simulink model "part2"  (R2020a)
settings: Solver=ode23t  StartTime=0.0  StopTime=10  FixedStep=0.001  MaxStep=0.001  RelTol=1e-20
values from neighbouring files (symbols this model uses):
  mu = 1/82.45    (= 0.0121285627653)    [part1_sim.m]
  mu_star = 1 - mu    (= 0.987871437235)    [part1_sim.m]
settings Model: Creator=Ataka  LastModifiedBy=Ataka

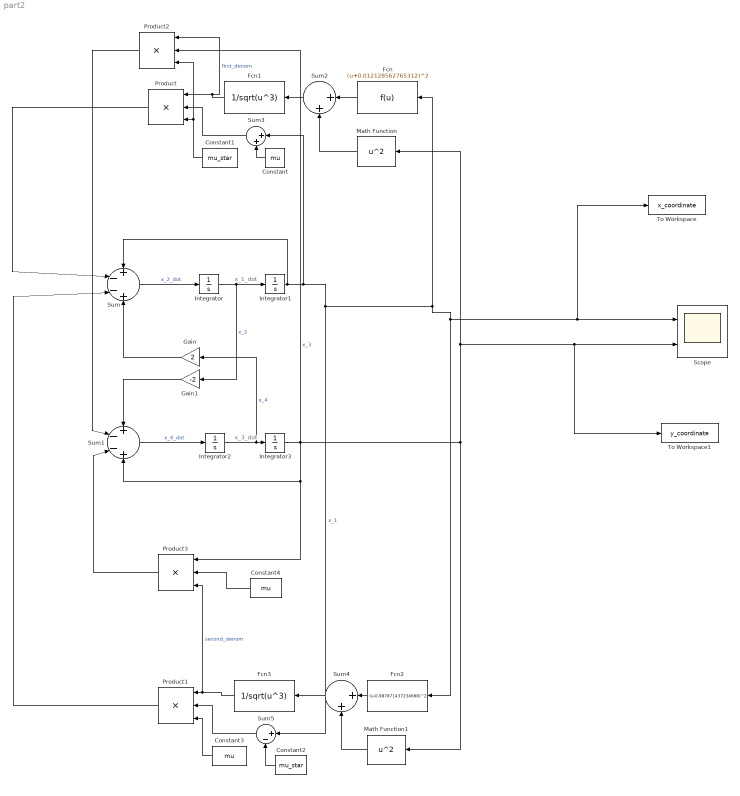
== system part2 ==
  note: x_1_dot
  note: x_3_dot
  Constant : Constant  Value=mu
  Constant1 : Constant  Value=mu_star
  Constant2 : Constant  Value=mu_star
  Constant3 : Constant  Value=mu
  Constant4 : Constant  Value=mu
  Fcn : Fcn  Expr=(u+0.012128562765312)^2
  Fcn1 : Fcn  Expr=1/sqrt(u^3)
  Fcn2 : Fcn  Expr=(u-0.987871437234688)^2
  Fcn3 : Fcn  Expr=1/sqrt(u^3)
  Gain : Gain  Gain=2
  Gain1 : Gain  Gain=-2
  Integrator : Integrator
  Integrator1 : Integrator  InitialCondition=1.2
  Integrator2 : Integrator  InitialCondition=-1.0494
  Integrator3 : Integrator
  Math Function : Math  Operator=square  SaturateOnIntegerOverflow=on
  Math Function1 : Math  Operator=square  SaturateOnIntegerOverflow=on
  Product{,1..3} (4 alike) : Product  Inputs=3
  Scope : Scope  NumInputPorts=2
  Sum : Sum  Inputs=+--+
  Sum1 : Sum  Inputs=+--+
  Sum2 : Sum  Inputs=|++
  Sum3 : Sum  Inputs=|++
  Sum4 : Sum  Inputs=|++
  Sum5 : Sum  Inputs=|+-
  To Workspace : ToWorkspace  VariableName=x_coordinate  SaveFormat=Timeseries  SampleTime=-1
  To Workspace1 : ToWorkspace  VariableName=y_coordinate  SaveFormat=Timeseries  SampleTime=-1
  wires:
  Sum/1 -> Integrator/1  "x_2_dot"
  Integrator/1 -> Gain1/1, Integrator1/1  "x_2"
  Integrator1/1 -> Sum3/1, Fcn/1, Fcn2/1, To Workspace/1, Scope/1, Sum5/1, Sum/1  "x_1"
  Integrator3/1 -> Product3/1, Sum1/4, Math Function/1, To Workspace1/1, Scope/2, Math Function1/1, Product2/2  "x_3"
  Integrator2/1 -> Gain/1, Integrator3/1  "x_4"
  Sum1/1 -> Integrator2/1  "x_4_dot"
  Gain1/1 -> Sum1/1
  Fcn/1 -> Sum2/1
  Math Function/1 -> Sum2/2
  Sum2/1 -> Fcn1/1
  Fcn1/1 -> Product/1, Product2/1  "first_denom"
  Constant/1 -> Sum3/2
  Sum3/1 -> Product/2
  Constant1/1 -> Product2/3, Product/3
  Gain/1 -> Sum/4
  Product/1 -> Sum/2
  Math Function1/1 -> Sum4/2
  Fcn2/1 -> Sum4/1
  Constant3/1 -> Product1/3
  Fcn3/1 -> Product3/3, Product1/1  "second_denom"
  Sum5/1 -> Product1/2
  Sum4/1 -> Fcn3/1
  Constant2/1 -> Sum5/2
  Product1/1 -> Sum/3
  Product2/1 -> Sum1/2
  Constant4/1 -> Product3/2
  Product3/1 -> Sum1/3
